simulink model "Q1"  (R2024b)
settings: Solver=VariableStepAuto  StartTime=0.0  StopTime=15  RelTol=1e-3
values from neighbouring files (symbols this model uses):
  c = 0.3    [Assignment_5.m]
  g = 9.81    [Assignment_5.m]
  m = 70    [Assignment_5.m]
settings Model: Creator=User  LastModifiedBy=User

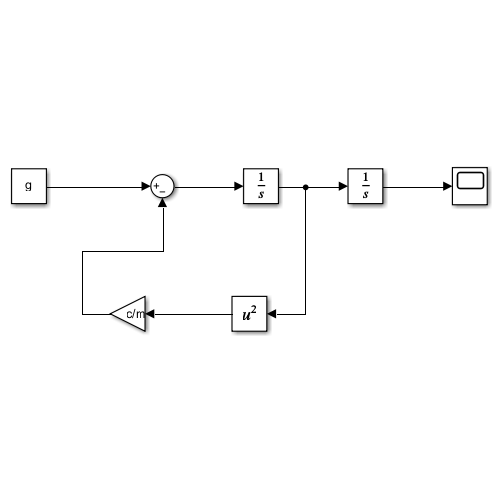
[thumbnail: Simulink's stored preview of the top-level diagram]
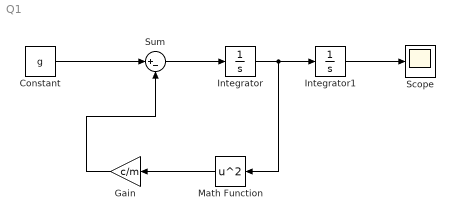
== system Q1 ==
  Constant : Constant  Value=g
  Gain : Gain  Gain=c/m
  Integrator : Integrator
  Integrator1 : Integrator
  Math Function : Math  Operator=square
  Scope : Scope
  Sum : Sum  Inputs=|+-
  wires:
  Constant/1 -> Sum/1
  Gain/1 -> Sum/2
  Sum/1 -> Integrator/1
  Integrator/1 -> Math Function/1, Integrator1/1
  Integrator1/1 -> Scope/1
  Math Function/1 -> Gain/1
